simulink model "HANcoder_E407_TTA_Template"  (R2018b)
settings: Solver=FixedStepDiscrete  StartTime=0.0  StopTime=1  FixedStep=0.01  RelTol=1e-3
PreLoadFcn:
  | librarySetup
  | eval([bdroot,'_startup']) %Calling [modelName]_startup.m
values from neighbouring files (symbols this model uses):
  basic_cycle_duration_bc0 = TM_Reset_Board   + COMP_duration    (= 212)    [HANcoder_E407_TTA_Controller_v3_5_startup.m]    (also in HANcoder_E407_TTA_Controller_v4_6_startup.m; HANcoder_E407_TTA_Controller_v4_7_startup.m; HANcoder_E407_TTA_Controller_v4_startup.m)
  basic_cycle_duration_bc1 = TM_Reset_Var_bc1 + COMP_duration    (= 288)    [HANcoder_E407_TTA_Controller_v3_5_startup.m]    (also in HANcoder_E407_TTA_Controller_v4_6_startup.m = 332; HANcoder_E407_TTA_Controller_v4_7_startup.m = 372; HANcoder_E407_TTA_Controller_v4_startup.m = 332)
  comm_delay_estimation1 = round(comm_delay_measured1*hardware_granularity/frequency_IRQ)    [HANcoder_E407_TTA_Controller_v3_5_startup.m]    (also in HANcoder_E407_TTA_Controller_v4_6_startup.m; HANcoder_E407_TTA_Controller_v4_7_startup.m; HANcoder_E407_TTA_Controller_v4_startup.m)
  comm_delay_estimation2 = round(comm_delay_measured2*hardware_granularity/frequency_IRQ)    [HANcoder_E407_TTA_Controller_v3_5_startup.m]    (also in HANcoder_E407_TTA_Controller_v4_6_startup.m; HANcoder_E407_TTA_Controller_v4_7_startup.m; HANcoder_E407_TTA_Controller_v4_startup.m)
  COMM_Period = 40    [HANcoder_E407_TTA_Controller_v3_5_startup.m]    (also in HANcoder_E407_TTA_Controller_v4_6_startup.m; HANcoder_E407_TTA_Controller_v4_7_startup.m; HANcoder_E407_TTA_Controller_v4_startup.m)
  COMM_Phase1 = Simulink.Parameter    [HANcoder_E407_TTA_Controller_v3_5_startup.m]    (also in HANcoder_E407_TTA_Controller_v4_6_startup.m; HANcoder_E407_TTA_Controller_v4_7_startup.m; HANcoder_E407_TTA_Controller_v4_startup.m)
  COMM_Phase2 = Simulink.Parameter    [HANcoder_E407_TTA_Controller_v3_5_startup.m]    (also in HANcoder_E407_TTA_Controller_v4_6_startup.m; HANcoder_E407_TTA_Controller_v4_7_startup.m; HANcoder_E407_TTA_Controller_v4_startup.m)
  COMM_Phase_init1 = Simulink.Parameter    [HANcoder_E407_TTA_Controller_v3_5_startup.m]    (also in HANcoder_E407_TTA_Controller_v4_6_startup.m; HANcoder_E407_TTA_Controller_v4_7_startup.m; HANcoder_E407_TTA_Controller_v4_startup.m)
  COMM_Phase_init2 = Simulink.Parameter    [HANcoder_E407_TTA_Controller_v3_5_startup.m]    (also in HANcoder_E407_TTA_Controller_v4_6_startup.m; HANcoder_E407_TTA_Controller_v4_7_startup.m; HANcoder_E407_TTA_Controller_v4_startup.m)
  COMP_duration = 4    [HANcoder_E407_TTA_Controller_v3_5_startup.m]    (also in HANcoder_E407_TTA_Controller_v4_6_startup.m; HANcoder_E407_TTA_Controller_v4_7_startup.m; HANcoder_E407_TTA_Controller_v4_startup.m)
  Controller1_Board = 1    [HANcoder_E407_TTA_Controller_v3_5_startup.m]    (also in HANcoder_E407_TTA_Controller_v4_6_startup.m; HANcoder_E407_TTA_Controller_v4_7_startup.m; HANcoder_E407_TTA_Controller_v4_startup.m)
  Controller2_Board = 2    [HANcoder_E407_TTA_Controller_v3_5_startup.m]    (also in HANcoder_E407_TTA_Controller_v4_6_startup.m; HANcoder_E407_TTA_Controller_v4_7_startup.m; HANcoder_E407_TTA_Controller_v4_startup.m)
  Controller3_Board = 3    [HANcoder_E407_TTA_Controller_v3_5_startup.m]    (also in HANcoder_E407_TTA_Controller_v4_6_startup.m; HANcoder_E407_TTA_Controller_v4_7_startup.m; HANcoder_E407_TTA_Controller_v4_startup.m)
  frequency_IRQ = 100    [HANcoder_E407_2xCAN_TEST_startup.m]    (also in HANcoder_E407_TTA_Controller_v3_5_startup.m; HANcoder_E407_TTA_Controller_v4_6_startup.m; HANcoder_E407_TTA_Controller_v4_7_startup.m; HANcoder_E407_TTA_Controller_v4_startup.m)
  HANtuneOverride = Simulink.Parameter    [HANcoder_E407_2xCAN_TEST_startup.m]    (also in HANcoder_E407_TTA_Controller_v3_5_startup.m; HANcoder_E407_TTA_Controller_v4_6_startup.m; HANcoder_E407_TTA_Controller_v4_7_startup.m; HANcoder_E407_TTA_Controller_v4_startup.m)
  idle_time_init = basic_cycle_duration_bc0 + basic_cycle_duration_bc1    (= 500)    [HANcoder_E407_TTA_Controller_v3_5_startup.m]    (also in HANcoder_E407_TTA_Controller_v4_6_startup.m = 544; HANcoder_E407_TTA_Controller_v4_7_startup.m = 584; HANcoder_E407_TTA_Controller_v4_startup.m = 544)
  LA_Clock_Gr = 1    [HANcoder_E407_TTA_Controller_v3_5_startup.m]    (also in HANcoder_E407_TTA_Controller_v4_6_startup.m; HANcoder_E407_TTA_Controller_v4_7_startup.m; HANcoder_E407_TTA_Controller_v4_startup.m)
  LA_COMM_dly = 1    [HANcoder_E407_TTA_Controller_v3_5_startup.m]    (also in HANcoder_E407_TTA_Controller_v4_6_startup.m; HANcoder_E407_TTA_Controller_v4_7_startup.m; HANcoder_E407_TTA_Controller_v4_startup.m)
  LA_COMM_Err = 1    [HANcoder_E407_TTA_Controller_v3_5_startup.m]    (also in HANcoder_E407_TTA_Controller_v4_6_startup.m; HANcoder_E407_TTA_Controller_v4_7_startup.m; HANcoder_E407_TTA_Controller_v4_startup.m)
  LA_E_Desync = 1    [HANcoder_E407_TTA_Controller_v3_5_startup.m]    (also in HANcoder_E407_TTA_Controller_v4_6_startup.m; HANcoder_E407_TTA_Controller_v4_7_startup.m; HANcoder_E407_TTA_Controller_v4_startup.m)
  LA_MEX_Flag = 1    [HANcoder_E407_TTA_Controller_v3_5_startup.m]    (also in HANcoder_E407_TTA_Controller_v4_6_startup.m; HANcoder_E407_TTA_Controller_v4_7_startup.m; HANcoder_E407_TTA_Controller_v4_startup.m)
  LA_Task_Act = 1    [HANcoder_E407_TTA_Controller_v3_5_startup.m]    (also in HANcoder_E407_TTA_Controller_v4_6_startup.m; HANcoder_E407_TTA_Controller_v4_7_startup.m; HANcoder_E407_TTA_Controller_v4_startup.m)
  Master_Role = 1    [HANcoder_E407_TTA_Controller_v3_5_startup.m]    (also in HANcoder_E407_TTA_Controller_v4_6_startup.m; HANcoder_E407_TTA_Controller_v4_7_startup.m; HANcoder_E407_TTA_Controller_v4_startup.m)
  matrix_rows = 2    [HANcoder_E407_TTA_Controller_v3_5_startup.m]    (also in HANcoder_E407_TTA_Controller_v4_6_startup.m; HANcoder_E407_TTA_Controller_v4_7_startup.m; HANcoder_E407_TTA_Controller_v4_startup.m)
  max_desync = 15    [HANcoder_E407_TTA_Controller_v3_5_startup.m]    (also in HANcoder_E407_TTA_Controller_v4_6_startup.m; HANcoder_E407_TTA_Controller_v4_7_startup.m = 30; HANcoder_E407_TTA_Controller_v4_startup.m)
  max_num_msgs_CAN1 = 2^Tx_bit_number-1    (= 7)    [HANcoder_E407_TTA_Controller_v3_5_startup.m]    (also in HANcoder_E407_TTA_Controller_v4_6_startup.m = 15; HANcoder_E407_TTA_Controller_v4_7_startup.m = 15; HANcoder_E407_TTA_Controller_v4_startup.m)
  max_num_msgs_CAN2 = max_num_msgs_CAN1    (= 7)    [HANcoder_E407_TTA_Controller_v3_5_startup.m]    (also in HANcoder_E407_TTA_Controller_v4_6_startup.m = 15; HANcoder_E407_TTA_Controller_v4_7_startup.m = 15; HANcoder_E407_TTA_Controller_v4_startup.m)
  min_desync = (-1)*max_desync    (= -15)    [HANcoder_E407_TTA_Controller_v3_5_startup.m]    (also in HANcoder_E407_TTA_Controller_v4_6_startup.m; HANcoder_E407_TTA_Controller_v4_7_startup.m = -30; HANcoder_E407_TTA_Controller_v4_startup.m)
  OutControl1_ID = 23    [HANcoder_E407_TTA_Controller_v3_5_startup.m]    (also in HANcoder_E407_TTA_Controller_v4_6_startup.m; HANcoder_E407_TTA_Controller_v4_7_startup.m; HANcoder_E407_TTA_Controller_v4_startup.m)
  OutControl2_ID = 24    [HANcoder_E407_TTA_Controller_v3_5_startup.m]    (also in HANcoder_E407_TTA_Controller_v4_6_startup.m; HANcoder_E407_TTA_Controller_v4_7_startup.m; HANcoder_E407_TTA_Controller_v4_startup.m)
  OutEmulator_ID = 25    [HANcoder_E407_TTA_Controller_v3_5_startup.m]    (also in HANcoder_E407_TTA_Controller_v4_6_startup.m = 26; HANcoder_E407_TTA_Controller_v4_7_startup.m = 26; HANcoder_E407_TTA_Controller_v4_startup.m)
  script_run = Simulink.Parameter    [HANcoder_E407_TTA_Controller_v3_5_startup.m]    (also in HANcoder_E407_TTA_Controller_v4_6_startup.m; HANcoder_E407_TTA_Controller_v4_7_startup.m; HANcoder_E407_TTA_Controller_v4_startup.m)
  SensorValues_ID = 22    [HANcoder_E407_TTA_Controller_v3_5_startup.m]    (also in HANcoder_E407_TTA_Controller_v4_6_startup.m; HANcoder_E407_TTA_Controller_v4_7_startup.m; HANcoder_E407_TTA_Controller_v4_startup.m)
  SetValues_ID = 21    [HANcoder_E407_TTA_Controller_v3_5_startup.m]    (also in HANcoder_E407_TTA_Controller_v4_6_startup.m; HANcoder_E407_TTA_Controller_v4_7_startup.m; HANcoder_E407_TTA_Controller_v4_startup.m)
  Slave_Role = 2    [HANcoder_E407_TTA_Controller_v3_5_startup.m]    (also in HANcoder_E407_TTA_Controller_v4_6_startup.m; HANcoder_E407_TTA_Controller_v4_7_startup.m; HANcoder_E407_TTA_Controller_v4_startup.m)
  Sync_ID = 1    [HANcoder_E407_TTA_Controller_v3_5_startup.m]    (also in HANcoder_E407_TTA_Controller_v4_6_startup.m; HANcoder_E407_TTA_Controller_v4_7_startup.m; HANcoder_E407_TTA_Controller_v4_startup.m)
  TM_Check_Sync = TM_COMM_Sync   + COMM_duration    (= 40)    [HANcoder_E407_TTA_Controller_v3_5_startup.m]    (also in HANcoder_E407_TTA_Controller_v4_6_startup.m; HANcoder_E407_TTA_Controller_v4_7_startup.m; HANcoder_E407_TTA_Controller_v4_startup.m)
  TM_Check_TOuts = TM_Count_Vote3 + COMP_duration    (= 196)    [HANcoder_E407_TTA_Controller_v3_5_startup.m]    (also in HANcoder_E407_TTA_Controller_v4_6_startup.m; HANcoder_E407_TTA_Controller_v4_7_startup.m; HANcoder_E407_TTA_Controller_v4_startup.m)
  TM_Check_Vote1 = TM_COMM_Vote1  + COMM_duration    (= 92)    [HANcoder_E407_TTA_Controller_v3_5_startup.m]    (also in HANcoder_E407_TTA_Controller_v4_6_startup.m; HANcoder_E407_TTA_Controller_v4_7_startup.m; HANcoder_E407_TTA_Controller_v4_startup.m)
  TM_Check_Vote2 = TM_COMM_Vote2  + COMM_duration    (= 140)    [HANcoder_E407_TTA_Controller_v3_5_startup.m]    (also in HANcoder_E407_TTA_Controller_v4_6_startup.m; HANcoder_E407_TTA_Controller_v4_7_startup.m; HANcoder_E407_TTA_Controller_v4_startup.m)
  TM_Check_Vote3 = TM_COMM_Vote3  + COMM_duration    (= 188)    [HANcoder_E407_TTA_Controller_v3_5_startup.m]    (also in HANcoder_E407_TTA_Controller_v4_6_startup.m; HANcoder_E407_TTA_Controller_v4_7_startup.m; HANcoder_E407_TTA_Controller_v4_startup.m)
  TM_COMM_Sync = basic_cycle_start    (= 0)    [HANcoder_E407_TTA_Controller_v3_5_startup.m]    (also in HANcoder_E407_TTA_Controller_v4_6_startup.m; HANcoder_E407_TTA_Controller_v4_7_startup.m; HANcoder_E407_TTA_Controller_v4_startup.m)
  TM_COMM_Vote1 = TM_Vote_Dec    + COMP_duration    (= 52)    [HANcoder_E407_TTA_Controller_v3_5_startup.m]    (also in HANcoder_E407_TTA_Controller_v4_6_startup.m; HANcoder_E407_TTA_Controller_v4_7_startup.m; HANcoder_E407_TTA_Controller_v4_startup.m)
  TM_COMM_Vote2 = TM_Count_Vote1 + COMP_duration    (= 100)    [HANcoder_E407_TTA_Controller_v3_5_startup.m]    (also in HANcoder_E407_TTA_Controller_v4_6_startup.m; HANcoder_E407_TTA_Controller_v4_7_startup.m; HANcoder_E407_TTA_Controller_v4_startup.m)
  TM_COMM_Vote3 = TM_Count_Vote2 + COMP_duration    (= 148)    [HANcoder_E407_TTA_Controller_v3_5_startup.m]    (also in HANcoder_E407_TTA_Controller_v4_6_startup.m; HANcoder_E407_TTA_Controller_v4_7_startup.m; HANcoder_E407_TTA_Controller_v4_startup.m)
  TM_Count_Vote1 = TM_Check_Vote1 + COMP_duration    (= 96)    [HANcoder_E407_TTA_Controller_v3_5_startup.m]    (also in HANcoder_E407_TTA_Controller_v4_6_startup.m; HANcoder_E407_TTA_Controller_v4_7_startup.m; HANcoder_E407_TTA_Controller_v4_startup.m)
  TM_Count_Vote2 = TM_Check_Vote2 + COMP_duration    (= 144)    [HANcoder_E407_TTA_Controller_v3_5_startup.m]    (also in HANcoder_E407_TTA_Controller_v4_6_startup.m; HANcoder_E407_TTA_Controller_v4_7_startup.m; HANcoder_E407_TTA_Controller_v4_startup.m)
  TM_Count_Vote3 = TM_Check_Vote3 + COMP_duration    (= 192)    [HANcoder_E407_TTA_Controller_v3_5_startup.m]    (also in HANcoder_E407_TTA_Controller_v4_6_startup.m; HANcoder_E407_TTA_Controller_v4_7_startup.m; HANcoder_E407_TTA_Controller_v4_startup.m)
  TM_Data_bc0 = TM_COMM_Sync    (= 0)    [HANcoder_E407_TTA_Controller_v3_5_startup.m]    (also in HANcoder_E407_TTA_Controller_v4_6_startup.m; HANcoder_E407_TTA_Controller_v4_7_startup.m; HANcoder_E407_TTA_Controller_v4_startup.m)
  TM_Data_bc1 = TM_Data_bc0(1:4)    [HANcoder_E407_TTA_Controller_v3_5_startup.m]    (also in HANcoder_E407_TTA_Controller_v4_6_startup.m; HANcoder_E407_TTA_Controller_v4_7_startup.m; HANcoder_E407_TTA_Controller_v4_startup.m)
  TM_New_Master = TM_Check_TOuts + COMP_duration    (= 200)    [HANcoder_E407_TTA_Controller_v3_5_startup.m]    (also in HANcoder_E407_TTA_Controller_v4_6_startup.m; HANcoder_E407_TTA_Controller_v4_7_startup.m; HANcoder_E407_TTA_Controller_v4_startup.m)
  TM_Reset_Board = TM_Reset_Var   + COMP_duration    (= 208)    [HANcoder_E407_TTA_Controller_v3_5_startup.m]    (also in HANcoder_E407_TTA_Controller_v4_6_startup.m; HANcoder_E407_TTA_Controller_v4_7_startup.m; HANcoder_E407_TTA_Controller_v4_startup.m)
  TM_Reset_Var = TM_New_Master  + COMP_duration    (= 204)    [HANcoder_E407_TTA_Controller_v3_5_startup.m]    (also in HANcoder_E407_TTA_Controller_v4_6_startup.m; HANcoder_E407_TTA_Controller_v4_7_startup.m; HANcoder_E407_TTA_Controller_v4_startup.m)
  TM_Reset_Var_bc1 = TM_Check_Output_Emulator + COMP_duration    (= 284)    [HANcoder_E407_TTA_Controller_v3_5_startup.m]    (also in HANcoder_E407_TTA_Controller_v4_6_startup.m = 328; HANcoder_E407_TTA_Controller_v4_7_startup.m = 368; HANcoder_E407_TTA_Controller_v4_startup.m = 328)
  TM_Reset_Var_bc1_2 = TM_Reset_Var_bc1 + 2    (= 286)    [HANcoder_E407_TTA_Controller_v3_5_startup.m]    (also in HANcoder_E407_TTA_Controller_v4_6_startup.m = 330; HANcoder_E407_TTA_Controller_v4_7_startup.m = 370; HANcoder_E407_TTA_Controller_v4_startup.m = 330)
  TM_Type_bc0 = COMM    (= 0)    [HANcoder_E407_TTA_Controller_v3_5_startup.m]    (also in HANcoder_E407_TTA_Controller_v4_6_startup.m; HANcoder_E407_TTA_Controller_v4_7_startup.m; HANcoder_E407_TTA_Controller_v4_startup.m)
  TM_Type_bc1 = TM_Type_bc0(1:4)    [HANcoder_E407_TTA_Controller_v3_5_startup.m]    (also in HANcoder_E407_TTA_Controller_v4_6_startup.m; HANcoder_E407_TTA_Controller_v4_7_startup.m; HANcoder_E407_TTA_Controller_v4_startup.m)
  TM_Update_LT = TM_Check_Sync  + COMP_duration    (= 44)    [HANcoder_E407_TTA_Controller_v3_5_startup.m]    (also in HANcoder_E407_TTA_Controller_v4_6_startup.m; HANcoder_E407_TTA_Controller_v4_7_startup.m; HANcoder_E407_TTA_Controller_v4_startup.m)
  TM_Update_LT_2 = TM_Update_LT   + 2    (= 46)    [HANcoder_E407_TTA_Controller_v3_5_startup.m]    (also in HANcoder_E407_TTA_Controller_v4_6_startup.m; HANcoder_E407_TTA_Controller_v4_7_startup.m; HANcoder_E407_TTA_Controller_v4_startup.m)
  TM_Vote_Dec = TM_Update_LT   + COMP_duration    (= 48)    [HANcoder_E407_TTA_Controller_v3_5_startup.m]    (also in HANcoder_E407_TTA_Controller_v4_6_startup.m; HANcoder_E407_TTA_Controller_v4_7_startup.m; HANcoder_E407_TTA_Controller_v4_startup.m)
  Vote1_ID = 11    [HANcoder_E407_TTA_Controller_v3_5_startup.m]    (also in HANcoder_E407_TTA_Controller_v4_6_startup.m; HANcoder_E407_TTA_Controller_v4_7_startup.m; HANcoder_E407_TTA_Controller_v4_startup.m)
  Vote2_ID = 12    [HANcoder_E407_TTA_Controller_v3_5_startup.m]    (also in HANcoder_E407_TTA_Controller_v4_6_startup.m; HANcoder_E407_TTA_Controller_v4_7_startup.m; HANcoder_E407_TTA_Controller_v4_startup.m)
  Vote3_ID = 13    [HANcoder_E407_TTA_Controller_v3_5_startup.m]    (also in HANcoder_E407_TTA_Controller_v4_6_startup.m; HANcoder_E407_TTA_Controller_v4_7_startup.m; HANcoder_E407_TTA_Controller_v4_startup.m)
undefined symbols (not defined in the file or in its folder): A0, A1, A2, A3, A4, CON2, CON4, D10, D12, D13, D8, D9
libraries: hdlsllib x75, HANcoder_STM32_Target x28, simulink x3, simulink_extras x1
(part 3 of 13)

== system HANcoder_E407_TTA_Template/HANcoder STM32 Target - E407-STM32 algorithm/TTA CAN System/CAN2 Recieve/Update message buffers ==
  note: Logic Analyzer - DEBUG
      | Message received!
  note: CAN_Rx stop listening
  note: Received message
      | ready for processing
  note: Local time when the
      | message is received
  message : Inport  OutDataTypeStr=Bus: msg_buffer_type
  Enable : EnablePort
  AND : Logic  Inputs=3  IconShape=distinctive  AllPortsSameDT=off  OutDataTypeStr=boolean
  Bus Selector : BusSelector  OutputSignals=signal2,signal3,signal4,signal5,signal6,signal7,signal8,signal9
  Cast To Double : DataTypeConversion  OutDataTypeStr=double
  Constant : Constant  Value=Sync_ID
  Constant2 : Constant  Value=LA_COMM_dly
  Data Store Read : DataStoreRead  DataStoreName=RxID_CAN2
  Data Store Write : DataStoreWrite  DataStoreName=Toggle_Pin_A0
  Data Store Write1 : DataStoreWrite  DataStoreName=Msg_Rx_CAN2  DataStoreElements=Msg_Rx_CAN2.Buffer_1#Msg_Rx_CAN2.Buffer_2#Msg_Rx_CAN2.Buffer_3#Msg_Rx_CAN2.Buffer_4#Msg_Rx_CAN2.Buffer_5#Msg_Rx_CAN2.Buffer_6#Msg_Rx_CAN2.Buffer_7#Msg_Rx_CAN2.Buffer_8
  Data Store Write2 : DataStoreWrite  DataStoreName=New_Msg_Ready_CAN2
  Data Store Write5 : DataStoreWrite  DataStoreName=Rx_State_CAN2
  Data Store Write6 : DataStoreWrite  DataStoreName=Msg_Rx_Ticks_CAN2
  Equal : RelationalOperator  Operator===  OutDataTypeStr=boolean  RndMeth=Simplest
  Idle_State : Constant  Value=3  OutDataTypeStr=uint8
  Local_Time : DataStoreRead  DataStoreName=Local_Ticks
  Logic Analyzer - COMM delay measurement : Subsystem  TreatAsAtomicUnit=on
  SET : Constant  OutDataTypeStr=boolean
  Terminator : Terminator
  wires:
  Local_Time/1 -> Data Store Write6/1  "Rx_msg_ticks_CAN2"
  message/1 -> Bus Selector/1
  Idle_State/1 -> Data Store Write5/1
  Bus Selector/1 -> Cast To Double/1, Data Store Write1/1  "<signal2>"
  Bus Selector/2 -> Data Store Write1/2  "<signal3>"
  Bus Selector/3 -> Data Store Write1/3  "<signal4>"
  Bus Selector/4 -> Data Store Write1/4  "<signal5>"
  Bus Selector/5 -> Data Store Write1/5  "<signal6>"
  Bus Selector/6 -> Data Store Write1/6  "<signal7>"
  Bus Selector/7 -> Data Store Write1/7  "<signal8>"
  Bus Selector/8 -> Data Store Write1/8  "<signal9>"
  Cast To Double/1 -> Terminator/1  "Rx_temporal_msg_CAN2"
  AND/1 -> Logic Analyzer - COMM delay measurement/Enable
  SET/1 -> Data Store Write2/1, Data Store Write/1, AND/2
  Data Store Read/1 -> Equal/1
  Constant2/1 -> AND/1
  Equal/1 -> AND/3
  Constant/1 -> Equal/2

== system HANcoder_E407_TTA_Template/HANcoder STM32 Target - E407-STM32 algorithm/TTA CAN System/CAN2 Send/CAN send1 ==
  In1 : Inport
  In2 : Inport  Port=2
  In3 : Inport  Port=3
  In4 : Inport  Port=4
  In5 : Inport  Port=5
  In6 : Inport  Port=6
  In7 : Inport  Port=7
  In8 : Inport  Port=8
  In9 : Inport  Port=9
  S-Function : M-S-Function  FunctionName=sfcn_can_send  Parameters=tsamp, canBus, frameType, inputNumber, dataType, byteOrder
  wires:
  In1/1 -> S-Function/1
  In2/1 -> S-Function/2
  In3/1 -> S-Function/3
  In4/1 -> S-Function/4
  In5/1 -> S-Function/5
  In6/1 -> S-Function/6
  In7/1 -> S-Function/7
  In8/1 -> S-Function/8
  In9/1 -> S-Function/9

== system HANcoder_E407_TTA_Template/HANcoder STM32 Target - E407-STM32 algorithm/TTA CAN System/CAN2 Send/Logic Analyzer - COMM delay measurement ==
  note: Set
  Enable : EnablePort
  Constant2 : Constant
  Data Store Write2 : DataStoreWrite  DataStoreName=Toggle_Pin_D9
  wires:
  Constant2/1 -> Data Store Write2/1

== system HANcoder_E407_TTA_Template/HANcoder STM32 Target - E407-STM32 algorithm/TTA CAN System/Measure EXecution time/DEBUG - Toggle digital pin A3 ==
  note: Change pin state
  note: Toggle pin data stored
  Enable : EnablePort
  Constant : Constant  OutDataTypeStr=boolean
  Constant1 : Constant  Value=0  OutDataTypeStr=boolean
  Data Store Read : DataStoreRead  DataStoreName=A3_Pin_State
  Data Store Read1 : DataStoreRead  DataStoreName=A3_Pin_State
  Data Store Write1 : DataStoreWrite  DataStoreName=A3_Pin_State
  Digital Output1 : HANcoder_STM32_Target/STM32-E407/Digital Outputs/Digital Output  Tag=HANcoder_TARGET_STM32_E407  pinID=CON2 - A3  config=Open drain  tsamp=-1
      settings: SourceProductName=HANcoder STM32 Target
  Switch : Switch  Criteria=u2 > Threshold
  wires:
  Switch/1 -> Data Store Write1/1
  Data Store Read/1 -> Switch/2
  Constant/1 -> Switch/3
  Constant1/1 -> Switch/1
  Data Store Read1/1 -> Digital Output1/1

== system HANcoder_E407_TTA_Template/HANcoder STM32 Target - E407-STM32 algorithm/TTA CAN System/TTA System/Basic Cycle Increment ==
  note: Local Time Reset
  note: Basic cycle counter
  Enable : EnablePort
  Add : Sum
  Add1 : Sum  Inputs=+-
  Cast : DataTypeConversion  OutDataTypeStr=uint8
  Constant : Constant  Value=matrix_rows
  Data Store Read4 : DataStoreRead  DataStoreName=basic_cycle_count
  Data Store Read5 : DataStoreRead  DataStoreName=basic_cycle_count
  Data Store Write : DataStoreWrite  DataStoreName=Local_Ticks
  Data Store Write3 : DataStoreWrite  DataStoreName=basic_cycle_count
  Decrement : Constant  OutDataTypeStr=uint8
  Increment : Constant  OutDataTypeStr=uint8
  LessThanOrEqual : RelationalOperator  Operator=<  OutDataTypeStr=boolean  RndMeth=Simplest
  Reset : Constant  Value=0  OutDataTypeStr=uint16
  Switch : Switch  Criteria=u2 > Threshold
  wires:
  Switch/1 -> Data Store Write3/1  "bacic_cycle_s"
  Data Store Read5/1 -> LessThanOrEqual/1
  Add/1 -> Switch/1
  Increment/1 -> Add/2
  Data Store Read4/1 -> Add/1
  LessThanOrEqual/1 -> Switch/2
  Constant/1 -> Add1/1
  Reset/1 -> Cast/1, Data Store Write/1
  Decrement/1 -> Add1/2
  Add1/1 -> LessThanOrEqual/2
  Cast/1 -> Switch/3

== system HANcoder_E407_TTA_Template/HANcoder STM32 Target - E407-STM32 algorithm/TTA CAN System/TTA System/DEBUG - Toggle digital pin A0 ==
  note: Change pin state
  note: Reset condition
  note: Toggle pin data stored
  Enable : EnablePort
  Constant : Constant  OutDataTypeStr=boolean
  Constant1 : Constant  Value=0  OutDataTypeStr=boolean
  Constant2 : Constant  Value=0  OutDataTypeStr=boolean
  Data Store Read : DataStoreRead  DataStoreName=A0_Pin_State
  Data Store Read1 : DataStoreRead  DataStoreName=A0_Pin_State
  Data Store Write : DataStoreWrite  DataStoreName=Toggle_Pin_A0
  Data Store Write1 : DataStoreWrite  DataStoreName=A0_Pin_State
  Digital Output : HANcoder_STM32_Target/STM32-E407/Digital Outputs/Digital Output  Tag=HANcoder_TARGET_STM32_E407  pinID=CON2 - A0  config=Open drain  tsamp=-1
      settings: SourceProductName=HANcoder STM32 Target
  Switch : Switch  Criteria=u2 > Threshold
  wires:
  Switch/1 -> Data Store Write1/1
  Data Store Read/1 -> Switch/2
  Constant/1 -> Switch/3
  Constant1/1 -> Switch/1
  Constant2/1 -> Data Store Write/1
  Data Store Read1/1 -> Digital Output/1

== system HANcoder_E407_TTA_Template/HANcoder STM32 Target - E407-STM32 algorithm/TTA CAN System/TTA System/DEBUG - Toggle digital pin A1 ==
  note: Toggle pin data stored
  note: Reset condition
  note: Change pin state
  Enable : EnablePort
  Constant : Constant  OutDataTypeStr=boolean
  Constant1 : Constant  Value=0  OutDataTypeStr=boolean
  Constant2 : Constant  Value=0  OutDataTypeStr=boolean
  Data Store Read : DataStoreRead  DataStoreName=A1_Pin_State
  Data Store Read1 : DataStoreRead  DataStoreName=A1_Pin_State
  Data Store Write : DataStoreWrite  DataStoreName=Toggle_Pin_A1
  Data Store Write1 : DataStoreWrite  DataStoreName=A1_Pin_State
  Digital Output : HANcoder_STM32_Target/STM32-E407/Digital Outputs/Digital Output  Tag=HANcoder_TARGET_STM32_E407  pinID=CON2 - A1  config=Open drain  tsamp=-1
      settings: SourceProductName=HANcoder STM32 Target
  Switch : Switch  Criteria=u2 > Threshold
  wires:
  Data Store Read1/1 -> Digital Output/1
  Constant2/1 -> Data Store Write/1
  Constant1/1 -> Switch/1
  Constant/1 -> Switch/3
  Data Store Read/1 -> Switch/2
  Switch/1 -> Data Store Write1/1

== system HANcoder_E407_TTA_Template/HANcoder STM32 Target - E407-STM32 algorithm/TTA CAN System/TTA System/DEBUG - Toggle digital pin A2 ==
  note: Toggle pin data stored
  note: Change pin state
  Enable : EnablePort
  Constant : Constant  OutDataTypeStr=boolean
  Constant1 : Constant  Value=0  OutDataTypeStr=boolean
  Data Store Read : DataStoreRead  DataStoreName=A2_Pin_State
  Data Store Read1 : DataStoreRead  DataStoreName=A2_Pin_State
  Data Store Write1 : DataStoreWrite  DataStoreName=A2_Pin_State
  Digital Output : HANcoder_STM32_Target/STM32-E407/Digital Outputs/Digital Output  Tag=HANcoder_TARGET_STM32_E407  pinID=CON2 - A2  config=Open drain  tsamp=-1
      settings: SourceProductName=HANcoder STM32 Target
  Switch : Switch  Criteria=u2 > Threshold
  wires:
  Data Store Read1/1 -> Digital Output/1
  Constant1/1 -> Switch/1
  Constant/1 -> Switch/3
  Data Store Read/1 -> Switch/2
  Switch/1 -> Data Store Write1/1

== system HANcoder_E407_TTA_Template/HANcoder STM32 Target - E407-STM32 algorithm/TTA CAN System/TTA System/DEBUG - Toggle digital pin A4 ==
  note: Toggle pin data stored
  note: Change pin state
  Enable : EnablePort
  Constant : Constant  OutDataTypeStr=boolean
  Constant1 : Constant  Value=0  OutDataTypeStr=boolean
  Data Store Read : DataStoreRead  DataStoreName=A4_Pin_State
  Data Store Read1 : DataStoreRead  DataStoreName=A4_Pin_State
  Data Store Write1 : DataStoreWrite  DataStoreName=A4_Pin_State
  Digital Output : HANcoder_STM32_Target/STM32-E407/Digital Outputs/Digital Output  Tag=HANcoder_TARGET_STM32_E407  pinID=CON2 - A4  config=Open drain  tsamp=-1
      settings: SourceProductName=HANcoder STM32 Target
  Switch : Switch  Criteria=u2 > Threshold
  wires:
  Data Store Read1/1 -> Digital Output/1
  Constant1/1 -> Switch/1
  Constant/1 -> Switch/3
  Data Store Read/1 -> Switch/2
  Switch/1 -> Data Store Write1/1

== system HANcoder_E407_TTA_Template/HANcoder STM32 Target - E407-STM32 algorithm/TTA CAN System/TTA System/DEBUG - Toggle digital pin D10 ==
  note: Change pin state
  note: Toggle pin data stored
  note: Reset condition
  Enable : EnablePort
  Constant : Constant  OutDataTypeStr=boolean
  Constant1 : Constant  Value=0  OutDataTypeStr=boolean
  Constant2 : Constant  Value=0  OutDataTypeStr=boolean
  Data Store Read : DataStoreRead  DataStoreName=D10_Pin_State
  Data Store Read1 : DataStoreRead  DataStoreName=D10_Pin_State
  Data Store Write : DataStoreWrite  DataStoreName=Toggle_Pin_D10
  Data Store Write1 : DataStoreWrite  DataStoreName=D10_Pin_State
  Digital Output : HANcoder_STM32_Target/STM32-E407/Digital Outputs/Digital Output  Tag=HANcoder_TARGET_STM32_E407  pinID=CON4 - D10  config=Open drain  tsamp=-1
      settings: SourceProductName=HANcoder STM32 Target
  Switch : Switch  Criteria=u2 > Threshold
  wires:
  Switch/1 -> Data Store Write1/1
  Data Store Read/1 -> Switch/2
  Constant/1 -> Switch/3
  Constant1/1 -> Switch/1
  Data Store Read1/1 -> Digital Output/1
  Constant2/1 -> Data Store Write/1

== system HANcoder_E407_TTA_Template/HANcoder STM32 Target - E407-STM32 algorithm/TTA CAN System/TTA System/Initialization ==
  Enable : EnablePort  PropagateVarSize=During execution
  AND : Logic  IconShape=distinctive  AllPortsSameDT=off  OutDataTypeStr=boolean
  Board nr1 : Constant  Value=Controller1_Board
  Board nr2 : Constant  Value=Controller2_Board
  Board nr3 : Constant  Value=Controller3_Board
  Constant : Constant  Value=idle_time_init
  Data Store Memory : DataStoreMemory  DataStoreName=Initialization_Timeout  ReadBeforeWriteMsg=warning  WriteAfterWriteMsg=warning  WriteAfterReadMsg=warning  ShowAdditionalParam=off  OutDataTypeStr=boolean
  Data Store Memory1 : DataStoreMemory  DataStoreName=Delay_Counter  ReadBeforeWriteMsg=warning  WriteAfterWriteMsg=warning  WriteAfterReadMsg=warning  ShowAdditionalParam=off  OutDataTypeStr=double
  Data Store Read : DataStoreRead  DataStoreName=New_Msg_Ready_CAN1
  Data Store Read1 : DataStoreRead  DataStoreName=Initialization_Timeout
  Data Store Read2 : DataStoreRead  DataStoreName=New_Msg_Ready_CAN2
  Data Store Read3 : DataStoreRead  DataStoreName=Board_ID
  Data Store Read4 : DataStoreRead  DataStoreName=Board_ID
  Data Store Read5 : DataStoreRead  DataStoreName=Board_ID
  Data Store Write : DataStoreWrite  DataStoreName=Initialization_Timeout
  Data Store Write1 : DataStoreWrite  DataStoreName=Initialization_flag
  Delay : Subsystem
  Equal : RelationalOperator  Operator===  OutDataTypeStr=boolean  RndMeth=Simplest
  Equal1 : RelationalOperator  Operator===  OutDataTypeStr=boolean  RndMeth=Simplest
  Equal2 : RelationalOperator  Operator===  OutDataTypeStr=boolean  RndMeth=Simplest
  NOT : Logic  Operator=NOT  IconShape=distinctive  AllPortsSameDT=off  OutDataTypeStr=boolean
  OR : Logic  Operator=OR  IconShape=distinctive  AllPortsSameDT=off  OutDataTypeStr=boolean
  OR1 : Logic  Operator=OR  IconShape=distinctive  AllPortsSameDT=off  OutDataTypeStr=boolean
  OR2 : Logic  Operator=OR  Inputs=3  IconShape=distinctive  AllPortsSameDT=off  OutDataTypeStr=boolean
  RoleID and Global Time init : Subsystem  TreatAsAtomicUnit=on
  wires:
  Delay/1(Output) -> Data Store Write/1
  Constant/1 -> Delay/1(Input)
  NOT/1 -> Data Store Write1/1
  RoleID and Global Time init/1(Finish Initialization) -> NOT/1
  OR/1 -> RoleID and Global Time init/Enable
  Data Store Read1/1 -> AND/2, RoleID and Global Time init/1(Timeout Initialization)
  OR1/1 -> OR/2, RoleID and Global Time init/2(Reference message received)
  Data Store Read4/1 -> Equal/1
  Board nr1/1 -> Equal/2
  OR2/1 -> AND/1
  AND/1 -> OR/1
  Data Store Read/1 -> OR1/1
  Data Store Read2/1 -> OR1/2
  Equal/1 -> OR2/1
  Equal1/1 -> OR2/2
  Equal2/1 -> OR2/3
  Board nr2/1 -> Equal1/2
  Data Store Read3/1 -> Equal1/1
  Board nr3/1 -> Equal2/2
  Data Store Read5/1 -> Equal2/1

== system HANcoder_E407_TTA_Template/HANcoder STM32 Target - E407-STM32 algorithm/TTA CAN System/TTA System/LT_Update Desync_Positive ==
  note: Local Time Update with Positive Desync
      | This subsystem is only activated if we have to update
      | the local time with a positive desync. This is activated
      | at the end of the current Computational Task, so the
      | Local Time is updated until the tick before the next
      | Computational Task in the basic cycle. This way we
      | avoid missing tasks, as would happened when updating
      | the Local Time too quickly into the future.
  note: WARNING
      | TM_Type is currently defined as
      | COMM type 0
      | COMP type 1
  note: Constants bc0
  note: constants are defined in the _startup file
  note: Constants bc1
  Local Time : Inport
  Bacic_Cycle : Inport  Port=2
  Enable : EnablePort  PropagateVarSize=During execution
  Bus Selector : BusSelector  OutputSignals=signal1,signal2
  Bus Creator : BusCreator  Inputs=2
  Bus Creator1 : BusCreator  Inputs=2
  Constant : Constant  Value=TM_Data_bc0
  Constant1 : Constant  Value=TM_Type_bc0
  Constant2 : Constant  Value=COMM_Phase1
  Constant3 : Constant  Value=COMM_Phase2
  Constant4 : Constant  Value=TM_Data_bc1
  Constant5 : Constant  Value=TM_Type_bc1
  Constant6 : Constant  Value=COMM_Phase_init1
  Constant7 : Constant  Value=COMM_Phase_init2
  Constant8 : Constant  Value=0
  Equal : RelationalOperator  Operator===  OutDataTypeStr=boolean  RndMeth=Simplest
  Local Time Update with Positive Desync : Subsystem  TreatAsAtomicUnit=on
  MATLAB Function : MATLAB Function  TreatAsAtomicUnit=on
  Switch : Switch  Criteria=u2 > Threshold  AllowDiffInputSizes=on
  wires:
  MATLAB Function/1(result_time) -> Local Time Update with Positive Desync/1(Ticks until next COMP)
  Local Time/1 -> MATLAB Function/1(local_time)
  Constant8/1 -> Equal/2
  Bacic_Cycle/1 -> Equal/1
  Equal/1 -> Switch/2
  Constant/1 -> Bus Creator/1
  Constant1/1 -> Bus Creator/2
  Bus Creator/1 -> Switch/1
  Constant4/1 -> Bus Creator1/1
  Constant5/1 -> Bus Creator1/2
  Bus Creator1/1 -> Switch/3
  Switch/1 -> Bus Selector/1
  Bus Selector/1 -> MATLAB Function/2(TM_data)  "<signal1>"
  Bus Selector/2 -> MATLAB Function/3(TM_type)  "<signal2>"
  Constant3/1 -> MATLAB Function/7(phase2)
  Constant2/1 -> MATLAB Function/5(phase1)
  Constant6/1 -> MATLAB Function/4(phase_init1)
  Constant7/1 -> MATLAB Function/6(phase_init2)

== system HANcoder_E407_TTA_Template/HANcoder STM32 Target - E407-STM32 algorithm/TTA CAN System/TTA System/Logic Analyzer - COMM delay CAN1 - Rx ==
  note: Change pin state
  note: Reset
  Enable : EnablePort
  Constant : Constant  OutDataTypeStr=boolean
  Constant1 : Constant  Value=0  OutDataTypeStr=boolean
  Constant2 : Constant  Value=0
  Data Store Read : DataStoreRead  DataStoreName=D12_Pin_State
  Data Store Read1 : DataStoreRead  Priority=2  DataStoreName=D12_Pin_State
  Data Store Write1 : DataStoreWrite  Priority=1  DataStoreName=D12_Pin_State
  Data Store Write2 : DataStoreWrite  Priority=3  DataStoreName=Toggle_Pin_D12
  Digital Output : HANcoder_STM32_Target/STM32-E407/Digital Outputs/Digital Output  Tag=HANcoder_TARGET_STM32_E407  pinID=CON4 - D12  config=Open drain  tsamp=-1
      settings: SourceProductName=HANcoder STM32 Target
  Switch : Switch  Criteria=u2 > Threshold
  wires:
  Data Store Read/1 -> Switch/2
  Data Store Read1/1 -> Digital Output/1
  Constant1/1 -> Switch/1
  Constant/1 -> Switch/3
  Switch/1 -> Data Store Write1/1
  Constant2/1 -> Data Store Write2/1

== system HANcoder_E407_TTA_Template/HANcoder STM32 Target - E407-STM32 algorithm/TTA CAN System/TTA System/Logic Analyzer - COMM delay CAN1 - Tx ==
  note: Reset
  note: Change pin state
  Enable : EnablePort
  Constant : Constant  OutDataTypeStr=boolean
  Constant1 : Constant  Value=0  OutDataTypeStr=boolean
  Constant2 : Constant  Value=0
  Data Store Read : DataStoreRead  DataStoreName=D13_Pin_State
  Data Store Read1 : DataStoreRead  Priority=2  DataStoreName=D13_Pin_State
  Data Store Write1 : DataStoreWrite  Priority=1  DataStoreName=D13_Pin_State
  Data Store Write2 : DataStoreWrite  Priority=3  DataStoreName=Toggle_Pin_D13
  Digital Output : HANcoder_STM32_Target/STM32-E407/Digital Outputs/Digital Output  Tag=HANcoder_TARGET_STM32_E407  pinID=CON4 - D13  config=Open drain  tsamp=-1
      settings: SourceProductName=HANcoder STM32 Target
  Switch : Switch  Criteria=u2 > Threshold
  wires:
  Switch/1 -> Data Store Write1/1
  Constant/1 -> Switch/3
  Constant1/1 -> Switch/1
  Data Store Read1/1 -> Digital Output/1
  Data Store Read/1 -> Switch/2
  Constant2/1 -> Data Store Write2/1

== system HANcoder_E407_TTA_Template/HANcoder STM32 Target - E407-STM32 algorithm/TTA CAN System/TTA System/Logic Analyzer - COMM delay CAN2 - Rx ==
  note: Change pin state
  note: Reset
  Enable : EnablePort
  Constant : Constant  OutDataTypeStr=boolean
  Constant1 : Constant  Value=0  OutDataTypeStr=boolean
  Constant2 : Constant  Value=0
  Data Store Read : DataStoreRead  DataStoreName=D8_Pin_State
  Data Store Read1 : DataStoreRead  Priority=2  DataStoreName=D8_Pin_State
  Data Store Write1 : DataStoreWrite  Priority=1  DataStoreName=D8_Pin_State
  Data Store Write2 : DataStoreWrite  Priority=3  DataStoreName=Toggle_Pin_D8
  Digital Output : HANcoder_STM32_Target/STM32-E407/Digital Outputs/Digital Output  Tag=HANcoder_TARGET_STM32_E407  pinID=CON4 - D8  config=Open drain  tsamp=-1
      settings: SourceProductName=HANcoder STM32 Target
  Switch : Switch  Criteria=u2 > Threshold
  wires:
  Data Store Read/1 -> Switch/2
  Data Store Read1/1 -> Digital Output/1
  Constant1/1 -> Switch/1
  Constant/1 -> Switch/3
  Switch/1 -> Data Store Write1/1
  Constant2/1 -> Data Store Write2/1

== system HANcoder_E407_TTA_Template/HANcoder STM32 Target - E407-STM32 algorithm/TTA CAN System/TTA System/Logic Analyzer - COMM delay CAN2 - Tx ==
  note: Change pin state
  note: Reset
  Enable : EnablePort
  Constant : Constant  OutDataTypeStr=boolean
  Constant1 : Constant  Value=0  OutDataTypeStr=boolean
  Constant2 : Constant  Value=0
  Data Store Read : DataStoreRead  DataStoreName=D9_Pin_State
  Data Store Read1 : DataStoreRead  Priority=2  DataStoreName=D9_Pin_State
  Data Store Write1 : DataStoreWrite  Priority=1  DataStoreName=D9_Pin_State
  Data Store Write2 : DataStoreWrite  Priority=3  DataStoreName=Toggle_Pin_D9
  Digital Output : HANcoder_STM32_Target/STM32-E407/Digital Outputs/Digital Output  Tag=HANcoder_TARGET_STM32_E407  pinID=CON4 - D9  config=Open drain  tsamp=-1
      settings: SourceProductName=HANcoder STM32 Target
  Switch : Switch  Criteria=u2 > Threshold
  wires:
  Switch/1 -> Data Store Write1/1
  Constant/1 -> Switch/3
  Constant1/1 -> Switch/1
  Data Store Read1/1 -> Digital Output/1
  Data Store Read/1 -> Switch/2
  Constant2/1 -> Data Store Write2/1

== system HANcoder_E407_TTA_Template/HANcoder STM32 Target - E407-STM32 algorithm/TTA CAN System/TTA System/Matrix Cycle Manager ==
  note: Controller boards condition
  note: Output Send_Message
      | Send: 1
      | Do not send: 0
  note: Output Receive_Message
      | Receive: 1
      | Do not receive: 0
  note: Output Receive_Message
      | Receive: 1
      | Do not receive: 0
  note: Output Send_Message
      | Send: 1
      | Do not send: 0
  Enable : EnablePort  PropagateVarSize=During execution
  Constant : Constant  Value=Controller1_Board
  Constant1 : Constant  Value=Controller2_Board
  Constant2 : Constant  Value=Controller3_Board
  Controller Matrix Cycle : Subsystem
  Data Store Read : DataStoreRead  DataStoreName=Board_ID
  Data Store Read10 : DataStoreRead  DataStoreName=basic_cycle_count
  Equal : RelationalOperator  Operator===  OutDataTypeStr=boolean  RndMeth=Simplest
  Equal1 : RelationalOperator  Operator===  OutDataTypeStr=boolean  RndMeth=Simplest
  Equal2 : RelationalOperator  Operator===  OutDataTypeStr=boolean  RndMeth=Simplest
  OR : Logic  Operator=OR  Inputs=3  IconShape=distinctive  AllPortsSameDT=off  OutDataTypeStr=boolean
  Send_Message_CAN1 : Outport  OutputWhenDisabled=reset  InitialOutput=0
  Send_Message_CAN2 : Outport  Port=2  OutputWhenDisabled=reset  InitialOutput=0
  Receive_Message_CAN1 : Outport  Port=3  OutputWhenDisabled=reset  InitialOutput=0
  Receive_Message_CAN2 : Outport  Port=4  OutputWhenDisabled=reset  InitialOutput=0
  wires:
  Data Store Read10/1 -> Controller Matrix Cycle/1(basic_cycle)
  Constant/1 -> Equal/2
  Constant1/1 -> Equal1/2
  Constant2/1 -> Equal2/2
  Equal/1 -> OR/1
  Equal1/1 -> OR/2
  Equal2/1 -> OR/3
  Data Store Read/1 -> Equal2/1, Equal1/1, Equal/1
  OR/1 -> Controller Matrix Cycle/Enable
  Controller Matrix Cycle/4(Receive_CAN2) -> Receive_Message_CAN2/1
  Controller Matrix Cycle/3(Receive_CAN1) -> Receive_Message_CAN1/1
  Controller Matrix Cycle/2(Send_CAN2) -> Send_Message_CAN2/1
  Controller Matrix Cycle/1(Send_CAN1) -> Send_Message_CAN1/1

== system HANcoder_E407_TTA_Template/HANcoder STM32 Target - E407-STM32 algorithm/TTA CAN System/CAN1 Recieve/RxID_CAN/OutControl1_ID_CAN ==
  Enable : EnablePort
  CAN receive1 : Subsystem  Tag=HANcoder_TARGET_STM32_E407  AncestorBlock=HANcoder_STM32_Target/STM32-E407/CAN/CAN/CAN receive  mask(CAN receive){canBus=CAN 1, outputNumber=8, dataType=uint8, byteOrder=off, tsamp=-1}
      mask prompts: canBus "CAN channel"; outputNumber "Output ports"; dataType "Output datatype"; byteOrder "Byte order: Checked = MSB first, unchecked = LSB first."; tsamp "Sample time"
      mask help:
      | Function
      | ==========
      | Receive the newest message from the specified CAN channel.
      |
      | Parameters
      | ==========
      | CAN channel:             The CAN channel to send the message on.
      | Output ports:             The amount of output ports
      | Output datatype:       The datatype of the output ports
      | Byte order:                 Select MSB or LSB first
      | Sample time:              -1 or divisible by base sample time [seconds]
      |
      | Input
      | ==========
      | Port 1:                       CAN ID(uint32) in hexadecimal ie: hex2dec('0a')
      |
      | Output
      | ==========
      | Port 1:                       Checks for new message(int8)
      | Port 2..9                     Message data
      mask init:
      | sfcn_can_receive_mcb(canBus, outputNumber, dataType, byteOrder)
      settings: MoveFcn=drawLogos
      mask Help: web('sfcn_can_receive.html');
      mask TypeOptions canBus: CAN 1 | CAN 2
      mask TypeOptions dataType: int8 | uint8 | int16 | uint16 | int32 | uint32 | boolean
      mask Display:
      | fprintf('Receive on\nCAN %x', canBus);
      | port_label('output', 1, 'new');
      | port_label('input', 1, 'ID');patch([135 141 141],[8 14 2],[1 0 0]);patch([143 143 149],[14 2 8],[0 0 0.35]);
  Constant6 : Constant  Value=OutControl1_ID  OutDataTypeStr=uint32
  CAN_new : Outport  OutputWhenDisabled=reset  InitialOutput=0
  Out2 : Outport  Port=2  OutputWhenDisabled=reset  InitialOutput=0
  Out3 : Outport  Port=3  OutputWhenDisabled=reset  InitialOutput=0
  Out4 : Outport  Port=4  OutputWhenDisabled=reset  InitialOutput=0
  Out5 : Outport  Port=5  OutputWhenDisabled=reset  InitialOutput=0
  Out6 : Outport  Port=6  OutputWhenDisabled=reset  InitialOutput=0
  Out7 : Outport  Port=7  OutputWhenDisabled=reset  InitialOutput=0
  Out8 : Outport  Port=8  OutputWhenDisabled=reset  InitialOutput=0
  Out9 : Outport  Port=9  OutputWhenDisabled=reset  InitialOutput=0
  wires:
  CAN receive1/1(Out1) -> CAN_new/1
  CAN receive1/8(Out8) -> Out8/1
  CAN receive1/3(Out3) -> Out3/1
  CAN receive1/2(Out2) -> Out2/1
  CAN receive1/6(Out6) -> Out6/1
  CAN receive1/7(Out7) -> Out7/1
  CAN receive1/4(Out4) -> Out4/1
  CAN receive1/5(Out5) -> Out5/1
  CAN receive1/9(Out9) -> Out9/1
  Constant6/1 -> CAN receive1/1(In1)

== system HANcoder_E407_TTA_Template/HANcoder STM32 Target - E407-STM32 algorithm/TTA CAN System/CAN1 Recieve/RxID_CAN/OutControl2_ID_CAN ==
  Enable : EnablePort
  CAN receive1 : Subsystem  Tag=HANcoder_TARGET_STM32_E407  AncestorBlock=HANcoder_STM32_Target/STM32-E407/CAN/CAN/CAN receive  mask(CAN receive){canBus=CAN 1, outputNumber=8, dataType=uint8, byteOrder=off, tsamp=-1}
      mask prompts: canBus "CAN channel"; outputNumber "Output ports"; dataType "Output datatype"; byteOrder "Byte order: Checked = MSB first, unchecked = LSB first."; tsamp "Sample time"
      mask help:
      | Function
      | ==========
      | Receive the newest message from the specified CAN channel.
      |
      | Parameters
      | ==========
      | CAN channel:             The CAN channel to send the message on.
      | Output ports:             The amount of output ports
      | Output datatype:       The datatype of the output ports
      | Byte order:                 Select MSB or LSB first
      | Sample time:              -1 or divisible by base sample time [seconds]
      |
      | Input
      | ==========
      | Port 1:                       CAN ID(uint32) in hexadecimal ie: hex2dec('0a')
      |
      | Output
      | ==========
      | Port 1:                       Checks for new message(int8)
      | Port 2..9                     Message data
      mask init:
      | sfcn_can_receive_mcb(canBus, outputNumber, dataType, byteOrder)
      settings: MoveFcn=drawLogos
      mask Help: web('sfcn_can_receive.html');
      mask TypeOptions canBus: CAN 1 | CAN 2
      mask TypeOptions dataType: int8 | uint8 | int16 | uint16 | int32 | uint32 | boolean
      mask Display:
      | fprintf('Receive on\nCAN %x', canBus);
      | port_label('output', 1, 'new');
      | port_label('input', 1, 'ID');patch([135 141 141],[8 14 2],[1 0 0]);patch([143 143 149],[14 2 8],[0 0 0.35]);
  Constant7 : Constant  Value=OutControl2_ID  OutDataTypeStr=uint32
  CAN_new : Outport  OutputWhenDisabled=reset  InitialOutput=0
  Out2 : Outport  Port=2  OutputWhenDisabled=reset  InitialOutput=0
  Out3 : Outport  Port=3  OutputWhenDisabled=reset  InitialOutput=0
  Out4 : Outport  Port=4  OutputWhenDisabled=reset  InitialOutput=0
  Out5 : Outport  Port=5  OutputWhenDisabled=reset  InitialOutput=0
  Out6 : Outport  Port=6  OutputWhenDisabled=reset  InitialOutput=0
  Out7 : Outport  Port=7  OutputWhenDisabled=reset  InitialOutput=0
  Out8 : Outport  Port=8  OutputWhenDisabled=reset  InitialOutput=0
  Out9 : Outport  Port=9  OutputWhenDisabled=reset  InitialOutput=0
  wires:
  Constant7/1 -> CAN receive1/1(In1)
  CAN receive1/9(Out9) -> Out9/1
  CAN receive1/5(Out5) -> Out5/1
  CAN receive1/4(Out4) -> Out4/1
  CAN receive1/7(Out7) -> Out7/1
  CAN receive1/6(Out6) -> Out6/1
  CAN receive1/2(Out2) -> Out2/1
  CAN receive1/3(Out3) -> Out3/1
  CAN receive1/8(Out8) -> Out8/1
  CAN receive1/1(Out1) -> CAN_new/1

== system HANcoder_E407_TTA_Template/HANcoder STM32 Target - E407-STM32 algorithm/TTA CAN System/CAN1 Recieve/RxID_CAN/OutEmulator_ID_CAN ==
  Enable : EnablePort
  CAN receive1 : Subsystem  Tag=HANcoder_TARGET_STM32_E407  AncestorBlock=HANcoder_STM32_Target/STM32-E407/CAN/CAN/CAN receive  mask(CAN receive){canBus=CAN 1, outputNumber=8, dataType=uint8, byteOrder=off, tsamp=-1}
      mask prompts: canBus "CAN channel"; outputNumber "Output ports"; dataType "Output datatype"; byteOrder "Byte order: Checked = MSB first, unchecked = LSB first."; tsamp "Sample time"
      mask help:
      | Function
      | ==========
      | Receive the newest message from the specified CAN channel.
      |
      | Parameters
      | ==========
      | CAN channel:             The CAN channel to send the message on.
      | Output ports:             The amount of output ports
      | Output datatype:       The datatype of the output ports
      | Byte order:                 Select MSB or LSB first
      | Sample time:              -1 or divisible by base sample time [seconds]
      |
      | Input
      | ==========
      | Port 1:                       CAN ID(uint32) in hexadecimal ie: hex2dec('0a')
      |
      | Output
      | ==========
      | Port 1:                       Checks for new message(int8)
      | Port 2..9                     Message data
      mask init:
      | sfcn_can_receive_mcb(canBus, outputNumber, dataType, byteOrder)
      settings: MoveFcn=drawLogos
      mask Help: web('sfcn_can_receive.html');
      mask TypeOptions canBus: CAN 1 | CAN 2
      mask TypeOptions dataType: int8 | uint8 | int16 | uint16 | int32 | uint32 | boolean
      mask Display:
      | fprintf('Receive on\nCAN %x', canBus);
      | port_label('output', 1, 'new');
      | port_label('input', 1, 'ID');patch([135 141 141],[8 14 2],[1 0 0]);patch([143 143 149],[14 2 8],[0 0 0.35]);
  Constant8 : Constant  Value=OutEmulator_ID  OutDataTypeStr=uint32
  CAN_new : Outport  OutputWhenDisabled=reset  InitialOutput=0
  Out2 : Outport  Port=2  OutputWhenDisabled=reset  InitialOutput=0
  Out3 : Outport  Port=3  OutputWhenDisabled=reset  InitialOutput=0
  Out4 : Outport  Port=4  OutputWhenDisabled=reset  InitialOutput=0
  Out5 : Outport  Port=5  OutputWhenDisabled=reset  InitialOutput=0
  Out6 : Outport  Port=6  OutputWhenDisabled=reset  InitialOutput=0
  Out7 : Outport  Port=7  OutputWhenDisabled=reset  InitialOutput=0
  Out8 : Outport  Port=8  OutputWhenDisabled=reset  InitialOutput=0
  Out9 : Outport  Port=9  OutputWhenDisabled=reset  InitialOutput=0
  wires:
  CAN receive1/1(Out1) -> CAN_new/1
  CAN receive1/8(Out8) -> Out8/1
  CAN receive1/3(Out3) -> Out3/1
  CAN receive1/2(Out2) -> Out2/1
  CAN receive1/6(Out6) -> Out6/1
  CAN receive1/7(Out7) -> Out7/1
  CAN receive1/4(Out4) -> Out4/1
  CAN receive1/5(Out5) -> Out5/1
  CAN receive1/9(Out9) -> Out9/1
  Constant8/1 -> CAN receive1/1(In1)

== system HANcoder_E407_TTA_Template/HANcoder STM32 Target - E407-STM32 algorithm/TTA CAN System/CAN1 Recieve/RxID_CAN/SensorValues_ID_CAN ==
  Enable : EnablePort
  CAN receive1 : Subsystem  Tag=HANcoder_TARGET_STM32_E407  AncestorBlock=HANcoder_STM32_Target/STM32-E407/CAN/CAN/CAN receive  mask(CAN receive){canBus=CAN 1, outputNumber=8, dataType=uint8, byteOrder=off, tsamp=-1}
      mask prompts: canBus "CAN channel"; outputNumber "Output ports"; dataType "Output datatype"; byteOrder "Byte order: Checked = MSB first, unchecked = LSB first."; tsamp "Sample time"
      mask help:
      | Function
      | ==========
      | Receive the newest message from the specified CAN channel.
      |
      | Parameters
      | ==========
      | CAN channel:             The CAN channel to send the message on.
      | Output ports:             The amount of output ports
      | Output datatype:       The datatype of the output ports
      | Byte order:                 Select MSB or LSB first
      | Sample time:              -1 or divisible by base sample time [seconds]
      |
      | Input
      | ==========
      | Port 1:                       CAN ID(uint32) in hexadecimal ie: hex2dec('0a')
      |
      | Output
      | ==========
      | Port 1:                       Checks for new message(int8)
      | Port 2..9                     Message data
      mask init:
      | sfcn_can_receive_mcb(canBus, outputNumber, dataType, byteOrder)
      settings: MoveFcn=drawLogos
      mask Help: web('sfcn_can_receive.html');
      mask TypeOptions canBus: CAN 1 | CAN 2
      mask TypeOptions dataType: int8 | uint8 | int16 | uint16 | int32 | uint32 | boolean
      mask Display:
      | fprintf('Receive on\nCAN %x', canBus);
      | port_label('output', 1, 'new');
      | port_label('input', 1, 'ID');patch([135 141 141],[8 14 2],[1 0 0]);patch([143 143 149],[14 2 8],[0 0 0.35]);
  Constant5 : Constant  Value=SensorValues_ID  OutDataTypeStr=uint32
  CAN_new : Outport  OutputWhenDisabled=reset  InitialOutput=0
  Out2 : Outport  Port=2  OutputWhenDisabled=reset  InitialOutput=0
  Out3 : Outport  Port=3  OutputWhenDisabled=reset  InitialOutput=0
  Out4 : Outport  Port=4  OutputWhenDisabled=reset  InitialOutput=0
  Out5 : Outport  Port=5  OutputWhenDisabled=reset  InitialOutput=0
  Out6 : Outport  Port=6  OutputWhenDisabled=reset  InitialOutput=0
  Out7 : Outport  Port=7  OutputWhenDisabled=reset  InitialOutput=0
  Out8 : Outport  Port=8  OutputWhenDisabled=reset  InitialOutput=0
  Out9 : Outport  Port=9  OutputWhenDisabled=reset  InitialOutput=0
  wires:
  Constant5/1 -> CAN receive1/1(In1)
  CAN receive1/9(Out9) -> Out9/1
  CAN receive1/5(Out5) -> Out5/1
  CAN receive1/4(Out4) -> Out4/1
  CAN receive1/7(Out7) -> Out7/1
  CAN receive1/6(Out6) -> Out6/1
  CAN receive1/2(Out2) -> Out2/1
  CAN receive1/3(Out3) -> Out3/1
  CAN receive1/8(Out8) -> Out8/1
  CAN receive1/1(Out1) -> CAN_new/1
